simulink model "JoystickControl_v2"  (Simulink 7.8)
settings: Solver=ode45  StartTime=0.0  StopTime=inf  RelTol=1e-3
StopFcn:
  | PioneerStopMotion
undefined symbols (not defined in the file or in its folder): Dopey
libraries: vrlib x1
settings Model: Creator=Drone3  LastModifiedBy=Admin
settings DataIOCC: SignalLoggingSaveFormat=Dataset
settings OptimizationCC: ExpressionDepthLimit=128
settings CodeAppCC: CustomSymbolStrType=$N$R$M_T

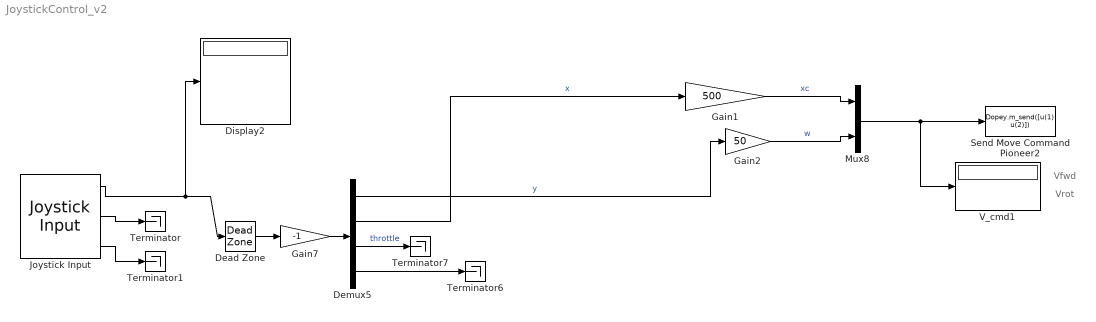
== system JoystickControl_v2 ==
  note: Vrot
  note: Vfwd
  Dead Zone : DeadZone  LowerValue=-.1  UpperValue=.12  SaturateOnIntegerOverflow=on
  Demux5 : Demux
  Display2 : Display
  Gain1 : Gain  Gain=500
  Gain2 : Gain  Gain=50
  Gain7 : Gain  Gain=-1
  Joystick Input : vrlib/Joystick Input  joyid=1  adjustports=on  forcefeed=off
  Mux8 : Mux  Inputs=2
  Send Move Command Pioneer2 : MATLABFcn  MATLABFcn=Dopey.m_send([u(1) u(2)])  OutputDimensions=0
  Terminator{,1,6..7} (4 alike) : Terminator
  V_cmd1 : Display
  wires:
  Demux5/2 -> Gain1/1  "x"
  Joystick Input/1 -> Dead Zone/1, Display2/1
  Gain1/1 -> Mux8/1  "xc"
  Gain2/1 -> Mux8/2  "w"
  Mux8/1 -> V_cmd1/1, Send Move Command Pioneer2/1
  Joystick Input/2 -> Terminator/1
  Joystick Input/3 -> Terminator1/1
  Demux5/3 -> Terminator7/1  "throttle"
  Demux5/4 -> Terminator6/1
  Demux5/1 -> Gain2/1  "y"
  Dead Zone/1 -> Gain7/1
  Gain7/1 -> Demux5/1
